simulink model "simul_P_control"  (Simulink 10.1)
settings: Solver=ode4  StartTime=0.0  StopTime=500  FixedStep=0.1  RelTol=1e-3  EnableMultiTasking=on
StartFcn:
  | clear all
values from neighbouring files (symbols this model uses):
  tau = M1.Td    [ident_via_contsid.m]    (also in test_your_model.m)
libraries: simulink x1
settings Model: Creator=johnh  LastModifiedBy=bluem1u
settings DataIOCC: SaveFormat=Dataset
settings DebuggingCC: UnderspecifiedInitializationDetection=Simplified  MergeDetectMultiDrivingBlocksExec=error  PregeneratedLibrarySubsystemCodeDiagnostic=none
settings HardwareCC: ProdBitPerPointer=64  ProdBitPerSizeT=64  ProdBitPerPtrDiffT=64  ProdLargestAtomicFloat=Float  ProdIntDivRoundTo=Zero  ProdEndianess=LittleEndian  ProdWordSize=64  ProdHWDeviceType=Intel->x86-64 (Windows64)
settings ModelReferenceCC: PropagateSignalLabelsOutOfModel=on
settings GRTTargetCC: CombineOutputUpdateFcns=on  GRTInterface=off

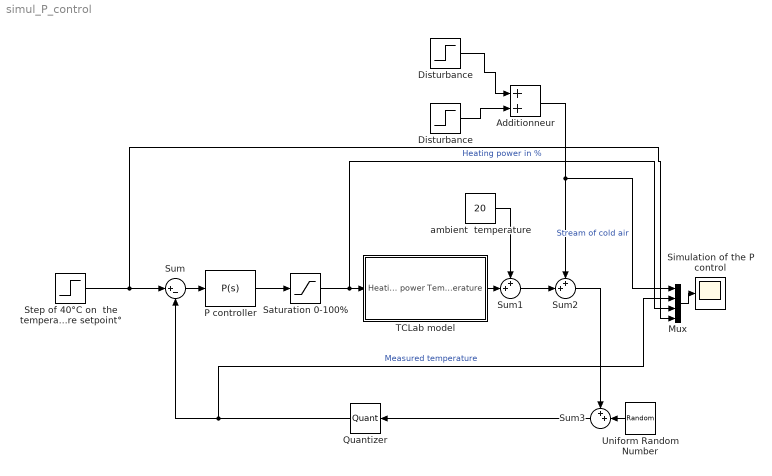
== system simul_P_control ==
  Additionneur : Sum
  Disturbance : Step  Time=300  After=-3  SampleTime=0
  "Disturbance " : Step  Time=320  After=+3  SampleTime=0
  Mux : Mux
  P controller : simulink/Continuous/PID Controller  Controller=P  Form=Parallel  TimeDomain=Continuous-time  UseExternalTs=off  SampleTime=-1  IntegratorMethod=Forward Euler  FilterMethod=Forward Euler  ControllerParametersSource=internal  P=10  I=1  D=1  UseFilter=on  N=100  TunerSelectOption=Transfer Function Based (PID Tuner App)  InitialConditionSource=internal  InitialConditionForIntegrator=0  InitialConditionForFilter=0  DifferentiatorICPrevScaledInput=0  ExternalReset=none  TrackingMode=off  Kt=1  LimitOutput=on  UpperSaturationLimit=100  LowerSaturationLimit=0  LinearizeAsGain=on  AntiWindupMode=clamping  Kb=1  POutMin=[]  POutMax=[]  IOutMin=[]  IOutMax=[]  DOutMin=[]  DOutMax=[]  NOutMin=[]  NOutMax=[]  SumOutMin=[]  SumOutMax=[]  SaturationOutMin=[]  SaturationOutMax=[]  PParamMin=[]  PParamMax=[]  IParamMin=[]  IParamMax=[]  DParamMin=[]  DParamMax=[]  NParamMin=[]  NParamMax=[]  KbParamMin=[]  KbParamMax=[]  KtParamMin=[]  KtParamMax=[]  KbOutMin=[]  KbOutMax=[]  KtOutMin=[]  KtOutMax=[]  IntegratorOutMin=[]  IntegratorOutMax=[]  FilterOutMin=[]  FilterOutMax=[]  SumI1OutMin=[]  SumI1OutMax=[]  SumI2OutMin=[]  SumI2OutMax=[]  SumI3OutMin=[]  SumI3OutMax=[]  SumI4OutMin=[]  SumI4OutMax=[]  SumDOutMin=[]  SumDOutMax=[]  DifferentiatorOutMin=[]  DifferentiatorOutMax=[]  FilterDiffOutCoefMin=[]  FilterDiffOutCoefMax=[]  ReciprocalOutMin=[]  ReciprocalOutMax=[]  SumDenOutMin=[]  SumDenOutMax=[]  SumNumOutMin=[]  SumNumOutMax=[]  DivideOutMin=[]  DivideOutMax=[]  UdiffTsProdOutMin=[]  UdiffTsProdOutMax=[]  NTsProdOutMin=[]  NTsProdOutMax=[]  UintegralTsProdOutMin=[]  UintegralTsProdOutMax=[]  UngainTsProdOutMin=[]  UngainTsProdOutMax=[]  IntegratorContinuousStateAttributes=''  IntegratorStateMustResolveToSignalObject=off  IntegratorRTWStateStorageClass=Auto  FilterContinuousStateAttributes=''  FilterStateMustResolveToSignalObject=off  FilterRTWStateStorageClass=Auto  ParallelPVariant=InternalParameters  IdealPVariant=Disabled  IVariant=Disabled  DVariant=Disabled  IntegratorVariant=Disabled  SatVariant=Enabled  AWVariant=Disabled  PCopyVariant=Disabled  TRVariant=Disabled  FdbkBlocksVariant=Forward  IdealPFdbkVariant=Disabled  SatFdbkVariant=Disabled  DerivativeFilterVariant=Disabled  NVariant=Disabled  NCopyVariant=Disabled_SignalSpec  FilterICVariant=Disabled  IntegratorICVariant=Disabled  ExternalResetVariant=Disabled  TRSumVariant=Passthrough  SumFdbkVariant=Disabled  SumVariant=Passthrough_P  TsampFilterVariant=InternalTs  TsampNgainVariant=Passthrough  TsampIntegralVariant=Disabled_SignalSpec
  Quantizer : Quantizer
  Saturation 0-100% : Saturate  UpperLimit=100  LowerLimit=0
  Simulation of the P control : Scope
  Step of 40°C on  the temperature setpoint° : Step  Time=20  Before=20  After=40  SampleTime=0
  Sum : Sum  Inputs=|+-
  Sum1 : Sum  Inputs=++|
  Sum2 : Sum  Inputs=++|
  Sum3 : Sum  Inputs=++|
  TCLab model : Subsystem
  Uniform Random Number : UniformRandomNumber  Minimum=-0.8  Maximum=0.8  SampleTime=0.1
  "ambient  temperature " : Constant  Value=20
  wires:
  Mux/1 -> Simulation of the P control/1
  Step of 40°C on  the temperature setpoint°/1 -> Mux/4, Sum/1
  Sum/1 -> P controller/1
  "ambient  temperature "/1 -> Sum1/1
  TCLab model/1("Temperature ") -> Sum1/2
  Sum1/1 -> Sum2/2
  Sum2/1 -> Sum3/1
  Disturbance/1 -> Additionneur/1
  "Disturbance "/1 -> Additionneur/2
  Additionneur/1 -> Mux/1, Sum2/1  "Stream of cold air"
  Uniform Random Number/1 -> Sum3/2
  P controller/1 -> Saturation 0-100%/1
  Saturation 0-100%/1 -> TCLab model/1("Heating power "), Mux/3  "Heating power in %"
  Quantizer/1 -> Mux/2, Sum/2  "Measured temperature"
  Sum3/1 -> Quantizer/1

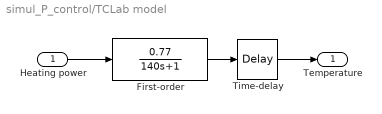
== system simul_P_control/TCLab model ==
  "Heating power " : Inport
  First-order : TransferFcn  Numerator=[0.77]  Denominator=[140 1]
  Time-delay : TransportDelay  DelayTime=tau
  "Temperature " : Outport  VectorParamsAs1DForOutWhenUnconnected=off
  wires:
  "Heating power "/1 -> First-order/1
  First-order/1 -> Time-delay/1
  Time-delay/1 -> "Temperature "/1
